simulink model "Ex2"  (R2020a)
settings: Solver=VariableStepAuto  StartTime=0.0  StopTime=10.0  RelTol=1e-3

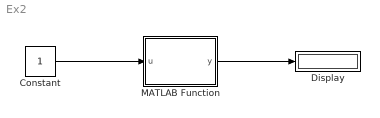
== system Ex2 ==
  Constant : Constant
  Display : Display
  MATLAB Function : MATLAB Function  TreatAsAtomicUnit=on
  wires:
  Constant/1 -> MATLAB Function/1(u)
  MATLAB Function/1(y) -> Display/1

== matlab function Ex2/MATLAB Function ==
  data: u input; y output
function y = fcn(u)

  if u>=1 u=u*u;
      else  u=u*u*u;
  end

y = u;
